simulink library "WARP_Blockset"  (Simulink 6.6)
libraries: xbsIndex_r4 x64
settings Model: Creator=murphpo  LastModifiedBy=Sid Gupta

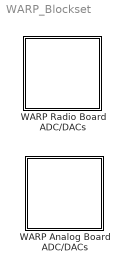
== system WARP_Blockset ==
  WARP Analog Board ADC/DACs : Subsystem
  WARP Radio Board ADC/DACs : Subsystem

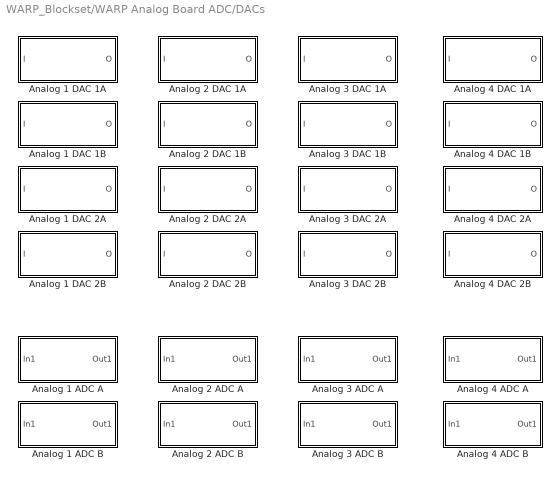
== system WARP_Blockset/WARP Analog Board ADC/DACs ==
  Analog 1 ADC A : Subsystem  mask{samp_period=1}
      mask prompts: samp_period "Sample Period"
      mask help: WARP Analog Board Slot 1 Analog-to-Digital Converter A
      mask Display: image(imread('WARP_Logo.jpg'))
  Analog 1 ADC B : Subsystem  mask{samp_period=1}
      mask prompts: samp_period "Sample Period"
      mask help: WARP Analog Board Slot 1 Analog-to-Digital Converter B
      mask Display: image(imread('WARP_Logo.jpg'))
  Analog 1 DAC 1A : Subsystem
      mask Description: WARP Analog Board Slot 1 Digital-to-Analog Converter 1A
      mask Display: image(imread('WARP_Logo.jpg'))
  Analog 1 DAC 1B : Subsystem
      mask Description: WARP Analog Board Slot 1 Digital-to-Analog Converter1B
      mask Display: image(imread('WARP_Logo.jpg'))
  Analog 1 DAC 2A : Subsystem
      mask Description: WARP Analog Board Slot 1 Digital-to-Analog Converter 2A
      mask Display: image(imread('WARP_Logo.jpg'))
  Analog 1 DAC 2B : Subsystem
      mask Description: WARP Analog Board Slot 1 Digital-to-Analog Converter 2B
      mask Display: image(imread('WARP_Logo.jpg'))
  Analog 2 ADC A : Subsystem  mask{samp_period=1}
      mask prompts: samp_period "Sample Period"
      mask help: WARP Analog Board Slot 2 Analog-to-Digital Converter A
      mask Display: image(imread('WARP_Logo.jpg'))
  Analog 2 ADC B : Subsystem  mask{samp_period=1}
      mask prompts: samp_period "Sample Period"
      mask help: WARP Analog Board Slot 2 Analog-to-Digital Converter B
      mask Display: image(imread('WARP_Logo.jpg'))
  Analog 2 DAC 1A : Subsystem
      mask Description: WARP Analog Board Slot 2 Digital-to-Analog Converter 1A
      mask Display: image(imread('WARP_Logo.jpg'))
  Analog 2 DAC 1B : Subsystem
      mask Description: WARP Analog Board Slot 2 Digital-to-Analog Converter1B
      mask Display: image(imread('WARP_Logo.jpg'))
  Analog 2 DAC 2A : Subsystem
      mask Description: WARP Analog Board Slot 2 Digital-to-Analog Converter 2A
      mask Display: image(imread('WARP_Logo.jpg'))
  Analog 2 DAC 2B : Subsystem
      mask Description: WARP Analog Board Slot 2 Digital-to-Analog Converter 2B
      mask Display: image(imread('WARP_Logo.jpg'))
  Analog 3 ADC A : Subsystem  mask{samp_period=1}
      mask prompts: samp_period "Sample Period"
      mask help: WARP Analog Board Slot 3 Analog-to-Digital Converter A
      mask Display: image(imread('WARP_Logo.jpg'))
  Analog 3 ADC B : Subsystem  mask{samp_period=1}
      mask prompts: samp_period "Sample Period"
      mask help: WARP Analog Board Slot 3 Analog-to-Digital Converter B
      mask Display: image(imread('WARP_Logo.jpg'))
  Analog 3 DAC 1A : Subsystem
      mask Description: WARP Analog Board Slot 3 Digital-to-Analog Converter 1A
      mask Display: image(imread('WARP_Logo.jpg'))
  Analog 3 DAC 1B : Subsystem
      mask Description: WARP Analog Board Slot 3 Digital-to-Analog Converter1B
      mask Display: image(imread('WARP_Logo.jpg'))
  Analog 3 DAC 2A : Subsystem
      mask Description: WARP Analog Board Slot 3 Digital-to-Analog Converter 2A
      mask Display: image(imread('WARP_Logo.jpg'))
  Analog 3 DAC 2B : Subsystem
      mask Description: WARP Analog Board Slot 3 Digital-to-Analog Converter 2B
      mask Display: image(imread('WARP_Logo.jpg'))
  Analog 4 ADC A : Subsystem  mask{samp_period=1}
      mask prompts: samp_period "Sample Period"
      mask help: WARP Analog Board Slot 4 Analog-to-Digital Converter A
      mask Display: image(imread('WARP_Logo.jpg'))
  Analog 4 ADC B : Subsystem  mask{samp_period=1}
      mask prompts: samp_period "Sample Period"
      mask help: WARP Analog Board Slot 4 Analog-to-Digital Converter B
      mask Display: image(imread('WARP_Logo.jpg'))
  Analog 4 DAC 1A : Subsystem
      mask Description: WARP Analog Board Slot 4 Digital-to-Analog Converter 1A
      mask Display: image(imread('WARP_Logo.jpg'))
  Analog 4 DAC 1B : Subsystem
      mask Description: WARP Analog Board Slot 4 Digital-to-Analog Converter1B
      mask Display: image(imread('WARP_Logo.jpg'))
  Analog 4 DAC 2A : Subsystem
      mask Description: WARP Analog Board Slot 4 Digital-to-Analog Converter 2A
      mask Display: image(imread('WARP_Logo.jpg'))
  Analog 4 DAC 2B : Subsystem
      mask Description: WARP Analog Board Slot 4 Digital-to-Analog Converter 2B
      mask Display: image(imread('WARP_Logo.jpg'))

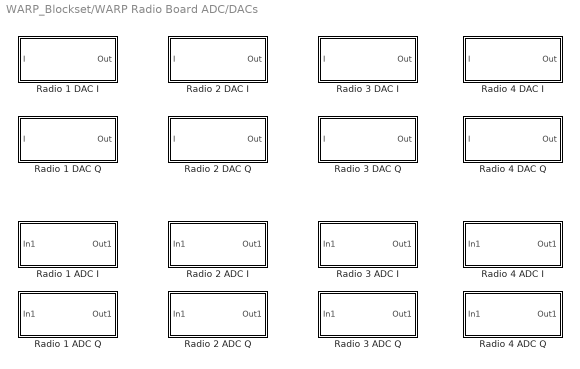
== system WARP_Blockset/WARP Radio Board ADC/DACs ==
  Radio 1 ADC I : Subsystem  mask{samp_period=1}
      mask prompts: samp_period "Sample Period"
      mask help: WARP Radio Board Slot 1 Analog-to-Digital Converter I-channel
      mask Display: image(imread('WARP_Logo.jpg'))
  Radio 1 ADC Q : Subsystem  mask{samp_period=1}
      mask prompts: samp_period "Sample Period"
      mask help: WARP Radio Board Slot 1 Analog-to-Digital Converter Q-channel
      mask Display: image(imread('WARP_Logo.jpg'))
  Radio 1 DAC I : Subsystem
      mask Description: WARP Radio Board Slot 1 Digital-to-Analog Converter I-channel
      mask Display: image(imread('WARP_Logo.jpg'))
  Radio 1 DAC Q : Subsystem
      mask Description: WARP Radio Board Slot 1 Digital-to-Analog Converter Q-channel
      mask Display: image(imread('WARP_Logo.jpg'))
  Radio 2 ADC I : Subsystem  mask{samp_period=1}
      mask prompts: samp_period "Sample Period"
      mask help: WARP Radio Board Slot 2 Analog-to-Digital Converter I-channel
      mask Display: image(imread('WARP_Logo.jpg'))
  Radio 2 ADC Q : Subsystem  mask{samp_period=1}
      mask prompts: samp_period "Sample Period"
      mask help: WARP Radio Board Slot 2 Analog-to-Digital Converter Q-channel
      mask Display: image(imread('WARP_Logo.jpg'))
  Radio 2 DAC I : Subsystem
      mask Description: WARP Radio Board Slot 2 Digital-to-Analog Converter I-channel
      mask Display: image(imread('WARP_Logo.jpg'))
  Radio 2 DAC Q : Subsystem
      mask Description: WARP Radio Board Slot 2 Digital-to-Analog Converter Q-channel
      mask Display: image(imread('WARP_Logo.jpg'))
  Radio 3 ADC I : Subsystem  mask{samp_period=1}
      mask prompts: samp_period "Sample Period"
      mask help: WARP Radio Board Slot 3 Analog-to-Digital Converter I-channel
      mask Display: image(imread('WARP_Logo.jpg'))
  Radio 3 ADC Q : Subsystem  mask{samp_period=1}
      mask prompts: samp_period "Sample Period"
      mask help: WARP Radio Board Slot 3 Analog-to-Digital Converter Q-channel
      mask Display: image(imread('WARP_Logo.jpg'))
  Radio 3 DAC I : Subsystem
      mask Description: WARP Radio Board Slot 3 Digital-to-Analog Converter I-channel
      mask Display: image(imread('WARP_Logo.jpg'))
  Radio 3 DAC Q : Subsystem
      mask Description: WARP Radio Board Slot 3 Digital-to-Analog Converter Q-channel
      mask Display: image(imread('WARP_Logo.jpg'))
  Radio 4 ADC I : Subsystem  mask{samp_period=1}
      mask prompts: samp_period "Sample Period"
      mask help: WARP Radio Board Slot 4 Analog-to-Digital Converter I-channel
      mask Display: image(imread('WARP_Logo.jpg'))
  Radio 4 ADC Q : Subsystem  mask{samp_period=1}
      mask prompts: samp_period "Sample Period"
      mask help: WARP Radio Board Slot 4 Analog-to-Digital Converter Q-channel
      mask Display: image(imread('WARP_Logo.jpg'))
  Radio 4 DAC I : Subsystem
      mask Description: WARP Radio Board Slot 4 Digital-to-Analog Converter I-channel
      mask Display: image(imread('WARP_Logo.jpg'))
  Radio 4 DAC Q : Subsystem
      mask Description: WARP Radio Board Slot 4 Digital-to-Analog Converter Q-channel
      mask Display: image(imread('WARP_Logo.jpg'))

== system WARP_Blockset/WARP Analog Board ADC/DACs/Analog 1 ADC A ==
  In1 : Inport
  analog1_adc_a : xbsIndex_r4/Gateway In  arith_type="Signed  (2's comp)"  n_bits=14  bin_pt=13  quantization="Round  (unbiased: +/- Inf)"  overflow=Flag as error  period=samp_period  dbl_ovrd=off  timing_constraint=None  locs_specified=off  LOCs={}  block_type=gatewayin
      settings: infoedit="Gateway in block.  Converts inputs of type Simulink integer, double and fixed point to  Xilinx fixed point type.<P><P>Hardware notes:  In hardware these blocks become top level input ports."  block_version=10.1.2
  Out1 : Outport
  wires:
  analog1_adc_a/1 -> Out1/1
  In1/1 -> analog1_adc_a/1

== system WARP_Blockset/WARP Analog Board ADC/DACs/Analog 1 ADC B ==
  In1 : Inport
  analog1_adc_b : xbsIndex_r4/Gateway In  arith_type="Signed  (2's comp)"  n_bits=14  bin_pt=13  quantization="Round  (unbiased: +/- Inf)"  overflow=Flag as error  period=samp_period  dbl_ovrd=off  timing_constraint=None  locs_specified=off  LOCs={}  block_type=gatewayin
      settings: infoedit="Gateway in block.  Converts inputs of type Simulink integer, double and fixed point to  Xilinx fixed point type.<P><P>Hardware notes:  In hardware these blocks become top level input ports."  block_version=10.1.2
  Out1 : Outport
  wires:
  In1/1 -> analog1_adc_b/1
  analog1_adc_b/1 -> Out1/1

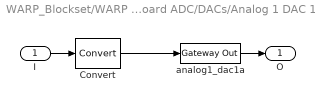
== system WARP_Blockset/WARP Analog Board ADC/DACs/Analog 1 DAC 1A ==
  I : Inport
  Convert : xbsIndex_r4/Convert  arith_type="Signed  (2's comp)"  n_bits=14  bin_pt=13  quantization=Truncate  overflow=Flag as error  latency=0  dbl_ovrd=off  pipeline=off  block_type=convert
      settings: block_version=10.1.2
  analog1_dac1a : xbsIndex_r4/Gateway Out  hdl_port=on  timing_constraint=None  locs_specified=off  LOCs={}  block_type=gatewayout
      settings: infoedit="Gateway out block.  Converts Xilinx fixed point inputs into ouputs of type Simulink integer, double, or fixed point.<P><P>Hardware notes:  In hardware these blocks become top level output ports or are discarded, depending on how they are configured."  block_version=10.1.2
  O : Outport
  wires:
  Convert/1 -> analog1_dac1a/1
  I/1 -> Convert/1
  analog1_dac1a/1 -> O/1

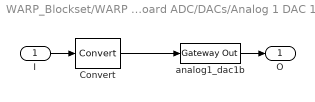
== system WARP_Blockset/WARP Analog Board ADC/DACs/Analog 1 DAC 1B ==
  I : Inport
  Convert : xbsIndex_r4/Convert  arith_type="Signed  (2's comp)"  n_bits=14  bin_pt=13  quantization=Truncate  overflow=Flag as error  latency=0  dbl_ovrd=off  pipeline=off  block_type=convert
      settings: block_version=10.1.2
  analog1_dac1b : xbsIndex_r4/Gateway Out  hdl_port=on  timing_constraint=None  locs_specified=off  LOCs={}  block_type=gatewayout
      settings: infoedit="Gateway out block.  Converts Xilinx fixed point inputs into ouputs of type Simulink integer, double, or fixed point.<P><P>Hardware notes:  In hardware these blocks become top level output ports or are discarded, depending on how they are configured."  block_version=10.1.2
  O : Outport
  wires:
  analog1_dac1b/1 -> O/1
  I/1 -> Convert/1
  Convert/1 -> analog1_dac1b/1

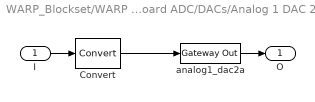
== system WARP_Blockset/WARP Analog Board ADC/DACs/Analog 1 DAC 2A ==
  I : Inport
  Convert : xbsIndex_r4/Convert  arith_type="Signed  (2's comp)"  n_bits=14  bin_pt=13  quantization=Truncate  overflow=Flag as error  latency=0  dbl_ovrd=off  pipeline=off  block_type=convert
      settings: block_version=10.1.2
  analog1_dac2a : xbsIndex_r4/Gateway Out  hdl_port=on  timing_constraint=None  locs_specified=off  LOCs={}  block_type=gatewayout
      settings: infoedit="Gateway out block.  Converts Xilinx fixed point inputs into ouputs of type Simulink integer, double, or fixed point.<P><P>Hardware notes:  In hardware these blocks become top level output ports or are discarded, depending on how they are configured."  block_version=10.1.2
  O : Outport
  wires:
  analog1_dac2a/1 -> O/1
  I/1 -> Convert/1
  Convert/1 -> analog1_dac2a/1

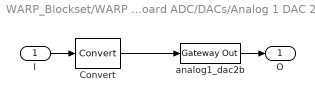
== system WARP_Blockset/WARP Analog Board ADC/DACs/Analog 1 DAC 2B ==
  I : Inport
  Convert : xbsIndex_r4/Convert  arith_type="Signed  (2's comp)"  n_bits=14  bin_pt=13  quantization=Truncate  overflow=Flag as error  latency=0  dbl_ovrd=off  pipeline=off  block_type=convert
      settings: block_version=10.1.2
  analog1_dac2b : xbsIndex_r4/Gateway Out  hdl_port=on  timing_constraint=None  locs_specified=off  LOCs={}  block_type=gatewayout
      settings: infoedit="Gateway out block.  Converts Xilinx fixed point inputs into ouputs of type Simulink integer, double, or fixed point.<P><P>Hardware notes:  In hardware these blocks become top level output ports or are discarded, depending on how they are configured."  block_version=10.1.2
  O : Outport
  wires:
  Convert/1 -> analog1_dac2b/1
  I/1 -> Convert/1
  analog1_dac2b/1 -> O/1

== system WARP_Blockset/WARP Analog Board ADC/DACs/Analog 2 ADC A ==
  In1 : Inport
  analog2_adc_a : xbsIndex_r4/Gateway In  arith_type="Signed  (2's comp)"  n_bits=14  bin_pt=13  quantization="Round  (unbiased: +/- Inf)"  overflow=Flag as error  period=samp_period  dbl_ovrd=off  timing_constraint=None  locs_specified=off  LOCs={}  block_type=gatewayin
      settings: infoedit="Gateway in block.  Converts inputs of type Simulink integer, double and fixed point to  Xilinx fixed point type.<P><P>Hardware notes:  In hardware these blocks become top level input ports."  block_version=10.1.2
  Out1 : Outport
  wires:
  In1/1 -> analog2_adc_a/1
  analog2_adc_a/1 -> Out1/1

== system WARP_Blockset/WARP Analog Board ADC/DACs/Analog 2 ADC B ==
  In1 : Inport
  analog2_adc_b : xbsIndex_r4/Gateway In  arith_type="Signed  (2's comp)"  n_bits=14  bin_pt=13  quantization="Round  (unbiased: +/- Inf)"  overflow=Flag as error  period=samp_period  dbl_ovrd=off  timing_constraint=None  locs_specified=off  LOCs={}  block_type=gatewayin
      settings: infoedit="Gateway in block.  Converts inputs of type Simulink integer, double and fixed point to  Xilinx fixed point type.<P><P>Hardware notes:  In hardware these blocks become top level input ports."  block_version=10.1.2
  Out1 : Outport
  wires:
  analog2_adc_b/1 -> Out1/1
  In1/1 -> analog2_adc_b/1

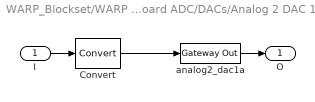
== system WARP_Blockset/WARP Analog Board ADC/DACs/Analog 2 DAC 1A ==
  I : Inport
  Convert : xbsIndex_r4/Convert  arith_type="Signed  (2's comp)"  n_bits=14  bin_pt=13  quantization=Truncate  overflow=Flag as error  latency=0  dbl_ovrd=off  pipeline=off  block_type=convert
      settings: block_version=10.1.2
  analog2_dac1a : xbsIndex_r4/Gateway Out  hdl_port=on  timing_constraint=None  locs_specified=off  LOCs={}  block_type=gatewayout
      settings: infoedit="Gateway out block.  Converts Xilinx fixed point inputs into ouputs of type Simulink integer, double, or fixed point.<P><P>Hardware notes:  In hardware these blocks become top level output ports or are discarded, depending on how they are configured."  block_version=10.1.2
  O : Outport
  wires:
  analog2_dac1a/1 -> O/1
  I/1 -> Convert/1
  Convert/1 -> analog2_dac1a/1

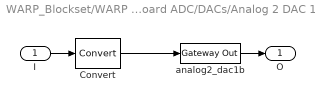
== system WARP_Blockset/WARP Analog Board ADC/DACs/Analog 2 DAC 1B ==
  I : Inport
  Convert : xbsIndex_r4/Convert  arith_type="Signed  (2's comp)"  n_bits=14  bin_pt=13  quantization=Truncate  overflow=Flag as error  latency=0  dbl_ovrd=off  pipeline=off  block_type=convert
      settings: block_version=10.1.2
  analog2_dac1b : xbsIndex_r4/Gateway Out  hdl_port=on  timing_constraint=None  locs_specified=off  LOCs={}  block_type=gatewayout
      settings: infoedit="Gateway out block.  Converts Xilinx fixed point inputs into ouputs of type Simulink integer, double, or fixed point.<P><P>Hardware notes:  In hardware these blocks become top level output ports or are discarded, depending on how they are configured."  block_version=10.1.2
  O : Outport
  wires:
  Convert/1 -> analog2_dac1b/1
  I/1 -> Convert/1
  analog2_dac1b/1 -> O/1

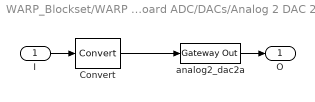
== system WARP_Blockset/WARP Analog Board ADC/DACs/Analog 2 DAC 2A ==
  I : Inport
  Convert : xbsIndex_r4/Convert  arith_type="Signed  (2's comp)"  n_bits=14  bin_pt=13  quantization=Truncate  overflow=Flag as error  latency=0  dbl_ovrd=off  pipeline=off  block_type=convert
      settings: block_version=10.1.2
  analog2_dac2a : xbsIndex_r4/Gateway Out  hdl_port=on  timing_constraint=None  locs_specified=off  LOCs={}  block_type=gatewayout
      settings: infoedit="Gateway out block.  Converts Xilinx fixed point inputs into ouputs of type Simulink integer, double, or fixed point.<P><P>Hardware notes:  In hardware these blocks become top level output ports or are discarded, depending on how they are configured."  block_version=10.1.2
  O : Outport
  wires:
  Convert/1 -> analog2_dac2a/1
  I/1 -> Convert/1
  analog2_dac2a/1 -> O/1

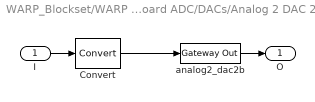
== system WARP_Blockset/WARP Analog Board ADC/DACs/Analog 2 DAC 2B ==
  I : Inport
  Convert : xbsIndex_r4/Convert  arith_type="Signed  (2's comp)"  n_bits=14  bin_pt=13  quantization=Truncate  overflow=Flag as error  latency=0  dbl_ovrd=off  pipeline=off  block_type=convert
      settings: block_version=10.1.2
  analog2_dac2b : xbsIndex_r4/Gateway Out  hdl_port=on  timing_constraint=None  locs_specified=off  LOCs={}  block_type=gatewayout
      settings: infoedit="Gateway out block.  Converts Xilinx fixed point inputs into ouputs of type Simulink integer, double, or fixed point.<P><P>Hardware notes:  In hardware these blocks become top level output ports or are discarded, depending on how they are configured."  block_version=10.1.2
  O : Outport
  wires:
  analog2_dac2b/1 -> O/1
  I/1 -> Convert/1
  Convert/1 -> analog2_dac2b/1

== system WARP_Blockset/WARP Analog Board ADC/DACs/Analog 3 ADC A ==
  In1 : Inport
  analog3_adc_a : xbsIndex_r4/Gateway In  arith_type="Signed  (2's comp)"  n_bits=14  bin_pt=13  quantization="Round  (unbiased: +/- Inf)"  overflow=Flag as error  period=samp_period  dbl_ovrd=off  timing_constraint=None  locs_specified=off  LOCs={}  block_type=gatewayin
      settings: infoedit="Gateway in block.  Converts inputs of type Simulink integer, double and fixed point to  Xilinx fixed point type.<P><P>Hardware notes:  In hardware these blocks become top level input ports."  block_version=10.1.2
  Out1 : Outport
  wires:
  In1/1 -> analog3_adc_a/1
  analog3_adc_a/1 -> Out1/1

== system WARP_Blockset/WARP Analog Board ADC/DACs/Analog 3 ADC B ==
  In1 : Inport
  analog3_adc_b : xbsIndex_r4/Gateway In  arith_type="Signed  (2's comp)"  n_bits=14  bin_pt=13  quantization="Round  (unbiased: +/- Inf)"  overflow=Flag as error  period=samp_period  dbl_ovrd=off  timing_constraint=None  locs_specified=off  LOCs={}  block_type=gatewayin
      settings: infoedit="Gateway in block.  Converts inputs of type Simulink integer, double and fixed point to  Xilinx fixed point type.<P><P>Hardware notes:  In hardware these blocks become top level input ports."  block_version=10.1.2
  Out1 : Outport
  wires:
  analog3_adc_b/1 -> Out1/1
  In1/1 -> analog3_adc_b/1

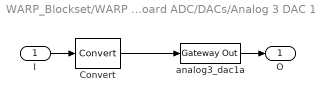
== system WARP_Blockset/WARP Analog Board ADC/DACs/Analog 3 DAC 1A ==
  I : Inport
  Convert : xbsIndex_r4/Convert  arith_type="Signed  (2's comp)"  n_bits=14  bin_pt=13  quantization=Truncate  overflow=Flag as error  latency=0  dbl_ovrd=off  pipeline=off  block_type=convert
      settings: block_version=10.1.2
  analog3_dac1a : xbsIndex_r4/Gateway Out  hdl_port=on  timing_constraint=None  locs_specified=off  LOCs={}  block_type=gatewayout
      settings: infoedit="Gateway out block.  Converts Xilinx fixed point inputs into ouputs of type Simulink integer, double, or fixed point.<P><P>Hardware notes:  In hardware these blocks become top level output ports or are discarded, depending on how they are configured."  block_version=10.1.2
  O : Outport
  wires:
  analog3_dac1a/1 -> O/1
  I/1 -> Convert/1
  Convert/1 -> analog3_dac1a/1

== system WARP_Blockset/WARP Analog Board ADC/DACs/Analog 3 DAC 1B ==
  I : Inport
  Convert : xbsIndex_r4/Convert  arith_type="Signed  (2's comp)"  n_bits=14  bin_pt=13  quantization=Truncate  overflow=Flag as error  latency=0  dbl_ovrd=off  pipeline=off  block_type=convert
      settings: block_version=10.1.2
  analog3_dac1b : xbsIndex_r4/Gateway Out  hdl_port=on  timing_constraint=None  locs_specified=off  LOCs={}  block_type=gatewayout
      settings: infoedit="Gateway out block.  Converts Xilinx fixed point inputs into ouputs of type Simulink integer, double, or fixed point.<P><P>Hardware notes:  In hardware these blocks become top level output ports or are discarded, depending on how they are configured."  block_version=10.1.2
  O : Outport
  wires:
  Convert/1 -> analog3_dac1b/1
  I/1 -> Convert/1
  analog3_dac1b/1 -> O/1

== system WARP_Blockset/WARP Analog Board ADC/DACs/Analog 3 DAC 2A ==
  I : Inport
  Convert : xbsIndex_r4/Convert  arith_type="Signed  (2's comp)"  n_bits=14  bin_pt=13  quantization=Truncate  overflow=Flag as error  latency=0  dbl_ovrd=off  pipeline=off  block_type=convert
      settings: block_version=10.1.2
  analog3_dac2a : xbsIndex_r4/Gateway Out  hdl_port=on  timing_constraint=None  locs_specified=off  LOCs={}  block_type=gatewayout
      settings: infoedit="Gateway out block.  Converts Xilinx fixed point inputs into ouputs of type Simulink integer, double, or fixed point.<P><P>Hardware notes:  In hardware these blocks become top level output ports or are discarded, depending on how they are configured."  block_version=10.1.2
  O : Outport
  wires:
  Convert/1 -> analog3_dac2a/1
  I/1 -> Convert/1
  analog3_dac2a/1 -> O/1

== system WARP_Blockset/WARP Analog Board ADC/DACs/Analog 3 DAC 2B ==
  I : Inport
  Convert : xbsIndex_r4/Convert  arith_type="Signed  (2's comp)"  n_bits=14  bin_pt=13  quantization=Truncate  overflow=Flag as error  latency=0  dbl_ovrd=off  pipeline=off  block_type=convert
      settings: block_version=10.1.2
  analog3_dac2b : xbsIndex_r4/Gateway Out  hdl_port=on  timing_constraint=None  locs_specified=off  LOCs={}  block_type=gatewayout
      settings: infoedit="Gateway out block.  Converts Xilinx fixed point inputs into ouputs of type Simulink integer, double, or fixed point.<P><P>Hardware notes:  In hardware these blocks become top level output ports or are discarded, depending on how they are configured."  block_version=10.1.2
  O : Outport
  wires:
  analog3_dac2b/1 -> O/1
  I/1 -> Convert/1
  Convert/1 -> analog3_dac2b/1

== system WARP_Blockset/WARP Analog Board ADC/DACs/Analog 4 ADC A ==
  In1 : Inport
  analog4_adc_a : xbsIndex_r4/Gateway In  arith_type="Signed  (2's comp)"  n_bits=14  bin_pt=13  quantization="Round  (unbiased: +/- Inf)"  overflow=Flag as error  period=samp_period  dbl_ovrd=off  timing_constraint=None  locs_specified=off  LOCs={}  block_type=gatewayin
      settings: infoedit="Gateway in block.  Converts inputs of type Simulink integer, double and fixed point to  Xilinx fixed point type.<P><P>Hardware notes:  In hardware these blocks become top level input ports."  block_version=10.1.2
  Out1 : Outport
  wires:
  In1/1 -> analog4_adc_a/1
  analog4_adc_a/1 -> Out1/1

== system WARP_Blockset/WARP Analog Board ADC/DACs/Analog 4 ADC B ==
  In1 : Inport
  analog4_adc_b : xbsIndex_r4/Gateway In  arith_type="Signed  (2's comp)"  n_bits=14  bin_pt=13  quantization="Round  (unbiased: +/- Inf)"  overflow=Flag as error  period=samp_period  dbl_ovrd=off  timing_constraint=None  locs_specified=off  LOCs={}  block_type=gatewayin
      settings: infoedit="Gateway in block.  Converts inputs of type Simulink integer, double and fixed point to  Xilinx fixed point type.<P><P>Hardware notes:  In hardware these blocks become top level input ports."  block_version=10.1.2
  Out1 : Outport
  wires:
  analog4_adc_b/1 -> Out1/1
  In1/1 -> analog4_adc_b/1

== system WARP_Blockset/WARP Analog Board ADC/DACs/Analog 4 DAC 1A ==
  I : Inport
  Convert : xbsIndex_r4/Convert  arith_type="Signed  (2's comp)"  n_bits=14  bin_pt=13  quantization=Truncate  overflow=Flag as error  latency=0  dbl_ovrd=off  pipeline=off  block_type=convert
      settings: block_version=10.1.2
  analog4_dac1a : xbsIndex_r4/Gateway Out  hdl_port=on  timing_constraint=None  locs_specified=off  LOCs={}  block_type=gatewayout
      settings: infoedit="Gateway out block.  Converts Xilinx fixed point inputs into ouputs of type Simulink integer, double, or fixed point.<P><P>Hardware notes:  In hardware these blocks become top level output ports or are discarded, depending on how they are configured."  block_version=10.1.2
  O : Outport
  wires:
  analog4_dac1a/1 -> O/1
  I/1 -> Convert/1
  Convert/1 -> analog4_dac1a/1

== system WARP_Blockset/WARP Analog Board ADC/DACs/Analog 4 DAC 1B ==
  I : Inport
  Convert : xbsIndex_r4/Convert  arith_type="Signed  (2's comp)"  n_bits=14  bin_pt=13  quantization=Truncate  overflow=Flag as error  latency=0  dbl_ovrd=off  pipeline=off  block_type=convert
      settings: block_version=10.1.2
  analog4_dac1b : xbsIndex_r4/Gateway Out  hdl_port=on  timing_constraint=None  locs_specified=off  LOCs={}  block_type=gatewayout
      settings: infoedit="Gateway out block.  Converts Xilinx fixed point inputs into ouputs of type Simulink integer, double, or fixed point.<P><P>Hardware notes:  In hardware these blocks become top level output ports or are discarded, depending on how they are configured."  block_version=10.1.2
  O : Outport
  wires:
  Convert/1 -> analog4_dac1b/1
  I/1 -> Convert/1
  analog4_dac1b/1 -> O/1

== system WARP_Blockset/WARP Analog Board ADC/DACs/Analog 4 DAC 2A ==
  I : Inport
  Convert : xbsIndex_r4/Convert  arith_type="Signed  (2's comp)"  n_bits=14  bin_pt=13  quantization=Truncate  overflow=Flag as error  latency=0  dbl_ovrd=off  pipeline=off  block_type=convert
      settings: block_version=10.1.2
  analog4_dac2a : xbsIndex_r4/Gateway Out  hdl_port=on  timing_constraint=None  locs_specified=off  LOCs={}  block_type=gatewayout
      settings: infoedit="Gateway out block.  Converts Xilinx fixed point inputs into ouputs of type Simulink integer, double, or fixed point.<P><P>Hardware notes:  In hardware these blocks become top level output ports or are discarded, depending on how they are configured."  block_version=10.1.2
  O : Outport
  wires:
  Convert/1 -> analog4_dac2a/1
  I/1 -> Convert/1
  analog4_dac2a/1 -> O/1

== system WARP_Blockset/WARP Analog Board ADC/DACs/Analog 4 DAC 2B ==
  I : Inport
  Convert : xbsIndex_r4/Convert  arith_type="Signed  (2's comp)"  n_bits=14  bin_pt=13  quantization=Truncate  overflow=Flag as error  latency=0  dbl_ovrd=off  pipeline=off  block_type=convert
      settings: block_version=10.1.2
  analog4_dac2b : xbsIndex_r4/Gateway Out  hdl_port=on  timing_constraint=None  locs_specified=off  LOCs={}  block_type=gatewayout
      settings: infoedit="Gateway out block.  Converts Xilinx fixed point inputs into ouputs of type Simulink integer, double, or fixed point.<P><P>Hardware notes:  In hardware these blocks become top level output ports or are discarded, depending on how they are configured."  block_version=10.1.2
  O : Outport
  wires:
  analog4_dac2b/1 -> O/1
  I/1 -> Convert/1
  Convert/1 -> analog4_dac2b/1

== system WARP_Blockset/WARP Radio Board ADC/DACs/Radio 1 ADC I ==
  In1 : Inport
  radio1_adc_I : xbsIndex_r4/Gateway In  arith_type="Signed  (2's comp)"  n_bits=14  bin_pt=13  quantization="Round  (unbiased: +/- Inf)"  overflow=Flag as error  period=samp_period  dbl_ovrd=off  timing_constraint=None  locs_specified=off  LOCs={}  block_type=gatewayin
      settings: infoedit="Gateway in block.  Converts inputs of type Simulink integer, double and fixed point to  Xilinx fixed point type.<P><P>Hardware notes:  In hardware these blocks become top level input ports."  block_version=10.1.2
  Out1 : Outport
  wires:
  In1/1 -> radio1_adc_I/1
  radio1_adc_I/1 -> Out1/1

== system WARP_Blockset/WARP Radio Board ADC/DACs/Radio 1 ADC Q ==
  In1 : Inport
  radio1_adc_Q : xbsIndex_r4/Gateway In  arith_type="Signed  (2's comp)"  n_bits=14  bin_pt=13  quantization="Round  (unbiased: +/- Inf)"  overflow=Flag as error  period=samp_period  dbl_ovrd=off  timing_constraint=None  locs_specified=off  LOCs={}  block_type=gatewayin
      settings: infoedit="Gateway in block.  Converts inputs of type Simulink integer, double and fixed point to  Xilinx fixed point type.<P><P>Hardware notes:  In hardware these blocks become top level input ports."  block_version=10.1.2
  Out1 : Outport
  wires:
  radio1_adc_Q/1 -> Out1/1
  In1/1 -> radio1_adc_Q/1

== system WARP_Blockset/WARP Radio Board ADC/DACs/Radio 1 DAC I ==
  I : Inport
  Convert : xbsIndex_r4/Convert  arith_type="Signed  (2's comp)"  n_bits=16  bin_pt=15  quantization=Truncate  overflow=Flag as error  latency=0  dbl_ovrd=off  pipeline=off  block_type=convert
      settings: block_version=10.1.2
  radio1_dac_I : xbsIndex_r4/Gateway Out  hdl_port=on  timing_constraint=None  locs_specified=off  LOCs={}  block_type=gatewayout
      settings: infoedit="Gateway out block.  Converts Xilinx fixed point inputs into ouputs of type Simulink integer, double, or fixed point.<P><P>Hardware notes:  In hardware these blocks become top level output ports or are discarded, depending on how they are configured."  block_version=10.1.2
  Out : Outport
  wires:
  Convert/1 -> radio1_dac_I/1
  I/1 -> Convert/1
  radio1_dac_I/1 -> Out/1

== system WARP_Blockset/WARP Radio Board ADC/DACs/Radio 1 DAC Q ==
  I : Inport
  Convert : xbsIndex_r4/Convert  arith_type="Signed  (2's comp)"  n_bits=16  bin_pt=15  quantization=Truncate  overflow=Flag as error  latency=0  dbl_ovrd=off  pipeline=off  block_type=convert
      settings: block_version=10.1.2
  radio1_dac_Q : xbsIndex_r4/Gateway Out  hdl_port=on  timing_constraint=None  locs_specified=off  LOCs={}  block_type=gatewayout
      settings: infoedit="Gateway out block.  Converts Xilinx fixed point inputs into ouputs of type Simulink integer, double, or fixed point.<P><P>Hardware notes:  In hardware these blocks become top level output ports or are discarded, depending on how they are configured."  block_version=10.1.2
  Out : Outport
  wires:
  radio1_dac_Q/1 -> Out/1
  I/1 -> Convert/1
  Convert/1 -> radio1_dac_Q/1

== system WARP_Blockset/WARP Radio Board ADC/DACs/Radio 2 ADC I ==
  In1 : Inport
  radio2_adc_I : xbsIndex_r4/Gateway In  arith_type="Signed  (2's comp)"  n_bits=14  bin_pt=13  quantization="Round  (unbiased: +/- Inf)"  overflow=Flag as error  period=samp_period  dbl_ovrd=off  timing_constraint=None  locs_specified=off  LOCs={}  block_type=gatewayin
      settings: infoedit="Gateway in block.  Converts inputs of type Simulink integer, double and fixed point to  Xilinx fixed point type.<P><P>Hardware notes:  In hardware these blocks become top level input ports."  block_version=10.1.2
  Out1 : Outport
  wires:
  radio2_adc_I/1 -> Out1/1
  In1/1 -> radio2_adc_I/1

== system WARP_Blockset/WARP Radio Board ADC/DACs/Radio 2 ADC Q ==
  In1 : Inport
  radio2_adc_Q : xbsIndex_r4/Gateway In  arith_type="Signed  (2's comp)"  n_bits=14  bin_pt=13  quantization="Round  (unbiased: +/- Inf)"  overflow=Flag as error  period=samp_period  dbl_ovrd=off  timing_constraint=None  locs_specified=off  LOCs={}  block_type=gatewayin
      settings: infoedit="Gateway in block.  Converts inputs of type Simulink integer, double and fixed point to  Xilinx fixed point type.<P><P>Hardware notes:  In hardware these blocks become top level input ports."  block_version=10.1.2
  Out1 : Outport
  wires:
  In1/1 -> radio2_adc_Q/1
  radio2_adc_Q/1 -> Out1/1

== system WARP_Blockset/WARP Radio Board ADC/DACs/Radio 2 DAC I ==
  I : Inport
  Convert : xbsIndex_r4/Convert  arith_type="Signed  (2's comp)"  n_bits=16  bin_pt=15  quantization=Truncate  overflow=Flag as error  latency=0  dbl_ovrd=off  pipeline=off  block_type=convert
      settings: block_version=10.1.2
  radio2_dac_I : xbsIndex_r4/Gateway Out  hdl_port=on  timing_constraint=None  locs_specified=off  LOCs={}  block_type=gatewayout
      settings: infoedit="Gateway out block.  Converts Xilinx fixed point inputs into ouputs of type Simulink integer, double, or fixed point.<P><P>Hardware notes:  In hardware these blocks become top level output ports or are discarded, depending on how they are configured."  block_version=10.1.2
  Out : Outport
  wires:
  radio2_dac_I/1 -> Out/1
  I/1 -> Convert/1
  Convert/1 -> radio2_dac_I/1

== system WARP_Blockset/WARP Radio Board ADC/DACs/Radio 2 DAC Q ==
  I : Inport
  Convert : xbsIndex_r4/Convert  arith_type="Signed  (2's comp)"  n_bits=16  bin_pt=15  quantization=Truncate  overflow=Flag as error  latency=0  dbl_ovrd=off  pipeline=off  block_type=convert
      settings: block_version=10.1.2
  radio2_dac_Q : xbsIndex_r4/Gateway Out  hdl_port=on  timing_constraint=None  locs_specified=off  LOCs={}  block_type=gatewayout
      settings: infoedit="Gateway out block.  Converts Xilinx fixed point inputs into ouputs of type Simulink integer, double, or fixed point.<P><P>Hardware notes:  In hardware these blocks become top level output ports or are discarded, depending on how they are configured."  block_version=10.1.2
  Out : Outport
  wires:
  Convert/1 -> radio2_dac_Q/1
  I/1 -> Convert/1
  radio2_dac_Q/1 -> Out/1

== system WARP_Blockset/WARP Radio Board ADC/DACs/Radio 3 ADC I ==
  In1 : Inport
  radio3_adc_I : xbsIndex_r4/Gateway In  arith_type="Signed  (2's comp)"  n_bits=14  bin_pt=13  quantization="Round  (unbiased: +/- Inf)"  overflow=Flag as error  period=samp_period  dbl_ovrd=off  timing_constraint=None  locs_specified=off  LOCs={}  block_type=gatewayin
      settings: infoedit="Gateway in block.  Converts inputs of type Simulink integer, double and fixed point to  Xilinx fixed point type.<P><P>Hardware notes:  In hardware these blocks become top level input ports."  block_version=10.1.2
  Out1 : Outport
  wires:
  radio3_adc_I/1 -> Out1/1
  In1/1 -> radio3_adc_I/1

== system WARP_Blockset/WARP Radio Board ADC/DACs/Radio 3 ADC Q ==
  In1 : Inport
  radio3_adc_Q : xbsIndex_r4/Gateway In  arith_type="Signed  (2's comp)"  n_bits=14  bin_pt=13  quantization="Round  (unbiased: +/- Inf)"  overflow=Flag as error  period=samp_period  dbl_ovrd=off  timing_constraint=None  locs_specified=off  LOCs={}  block_type=gatewayin
      settings: infoedit="Gateway in block.  Converts inputs of type Simulink integer, double and fixed point to  Xilinx fixed point type.<P><P>Hardware notes:  In hardware these blocks become top level input ports."  block_version=10.1.2
  Out1 : Outport
  wires:
  In1/1 -> radio3_adc_Q/1
  radio3_adc_Q/1 -> Out1/1

== system WARP_Blockset/WARP Radio Board ADC/DACs/Radio 3 DAC I ==
  I : Inport
  Convert : xbsIndex_r4/Convert  arith_type="Signed  (2's comp)"  n_bits=16  bin_pt=15  quantization=Truncate  overflow=Flag as error  latency=0  dbl_ovrd=off  pipeline=off  block_type=convert
      settings: block_version=10.1.2
  radio3_dac_I : xbsIndex_r4/Gateway Out  hdl_port=on  timing_constraint=None  locs_specified=off  LOCs={}  block_type=gatewayout
      settings: infoedit="Gateway out block.  Converts Xilinx fixed point inputs into ouputs of type Simulink integer, double, or fixed point.<P><P>Hardware notes:  In hardware these blocks become top level output ports or are discarded, depending on how they are configured."  block_version=10.1.2
  Out : Outport
  wires:
  Convert/1 -> radio3_dac_I/1
  I/1 -> Convert/1
  radio3_dac_I/1 -> Out/1

== system WARP_Blockset/WARP Radio Board ADC/DACs/Radio 3 DAC Q ==
  I : Inport
  Convert : xbsIndex_r4/Convert  arith_type="Signed  (2's comp)"  n_bits=16  bin_pt=15  quantization=Truncate  overflow=Flag as error  latency=0  dbl_ovrd=off  pipeline=off  block_type=convert
      settings: block_version=10.1.2
  radio3_dac_Q : xbsIndex_r4/Gateway Out  hdl_port=on  timing_constraint=None  locs_specified=off  LOCs={}  block_type=gatewayout
      settings: infoedit="Gateway out block.  Converts Xilinx fixed point inputs into ouputs of type Simulink integer, double, or fixed point.<P><P>Hardware notes:  In hardware these blocks become top level output ports or are discarded, depending on how they are configured."  block_version=10.1.2
  Out : Outport
  wires:
  radio3_dac_Q/1 -> Out/1
  I/1 -> Convert/1
  Convert/1 -> radio3_dac_Q/1

== system WARP_Blockset/WARP Radio Board ADC/DACs/Radio 4 ADC I ==
  In1 : Inport
  radio4_adc_I : xbsIndex_r4/Gateway In  arith_type="Signed  (2's comp)"  n_bits=14  bin_pt=13  quantization="Round  (unbiased: +/- Inf)"  overflow=Flag as error  period=samp_period  dbl_ovrd=off  timing_constraint=None  locs_specified=off  LOCs={}  block_type=gatewayin
      settings: infoedit="Gateway in block.  Converts inputs of type Simulink integer, double and fixed point to  Xilinx fixed point type.<P><P>Hardware notes:  In hardware these blocks become top level input ports."  block_version=10.1.2
  Out1 : Outport
  wires:
  radio4_adc_I/1 -> Out1/1
  In1/1 -> radio4_adc_I/1

== system WARP_Blockset/WARP Radio Board ADC/DACs/Radio 4 ADC Q ==
  In1 : Inport
  radio4_adc_Q : xbsIndex_r4/Gateway In  arith_type="Signed  (2's comp)"  n_bits=14  bin_pt=13  quantization="Round  (unbiased: +/- Inf)"  overflow=Flag as error  period=samp_period  dbl_ovrd=off  timing_constraint=None  locs_specified=off  LOCs={}  block_type=gatewayin
      settings: infoedit="Gateway in block.  Converts inputs of type Simulink integer, double and fixed point to  Xilinx fixed point type.<P><P>Hardware notes:  In hardware these blocks become top level input ports."  block_version=10.1.2
  Out1 : Outport
  wires:
  In1/1 -> radio4_adc_Q/1
  radio4_adc_Q/1 -> Out1/1

== system WARP_Blockset/WARP Radio Board ADC/DACs/Radio 4 DAC I ==
  I : Inport
  Convert : xbsIndex_r4/Convert  arith_type="Signed  (2's comp)"  n_bits=16  bin_pt=15  quantization=Truncate  overflow=Flag as error  latency=0  dbl_ovrd=off  pipeline=off  block_type=convert
      settings: block_version=10.1.2
  radio4_dac_I : xbsIndex_r4/Gateway Out  hdl_port=on  timing_constraint=None  locs_specified=off  LOCs={}  block_type=gatewayout
      settings: infoedit="Gateway out block.  Converts Xilinx fixed point inputs into ouputs of type Simulink integer, double, or fixed point.<P><P>Hardware notes:  In hardware these blocks become top level output ports or are discarded, depending on how they are configured."  block_version=10.1.2
  Out : Outport
  wires:
  radio4_dac_I/1 -> Out/1
  I/1 -> Convert/1
  Convert/1 -> radio4_dac_I/1

== system WARP_Blockset/WARP Radio Board ADC/DACs/Radio 4 DAC Q ==
  I : Inport
  Convert : xbsIndex_r4/Convert  arith_type="Signed  (2's comp)"  n_bits=16  bin_pt=15  quantization=Truncate  overflow=Flag as error  latency=0  dbl_ovrd=off  pipeline=off  block_type=convert
      settings: block_version=10.1.2
  radio4_dac_Q : xbsIndex_r4/Gateway Out  hdl_port=on  timing_constraint=None  locs_specified=off  LOCs={}  block_type=gatewayout
      settings: infoedit="Gateway out block.  Converts Xilinx fixed point inputs into ouputs of type Simulink integer, double, or fixed point.<P><P>Hardware notes:  In hardware these blocks become top level output ports or are discarded, depending on how they are configured."  block_version=10.1.2
  Out : Outport
  wires:
  Convert/1 -> radio4_dac_Q/1
  I/1 -> Convert/1
  radio4_dac_Q/1 -> Out/1
